simulink model "noloadwithcorrection"  (R2021a)
settings: Solver=VariableStepAuto  StartTime=0.0  StopTime=100  RelTol=1e-3
libraries: spsDCVoltageSourceLib x2, simulink x2, spsDCMachineLib x1, spsDiodeLib x1, spsGroundLib x1, spsIGBTDiodeLib x1, spspowerguiLib x1
settings Model: Creator=User  LastModifiedBy=User

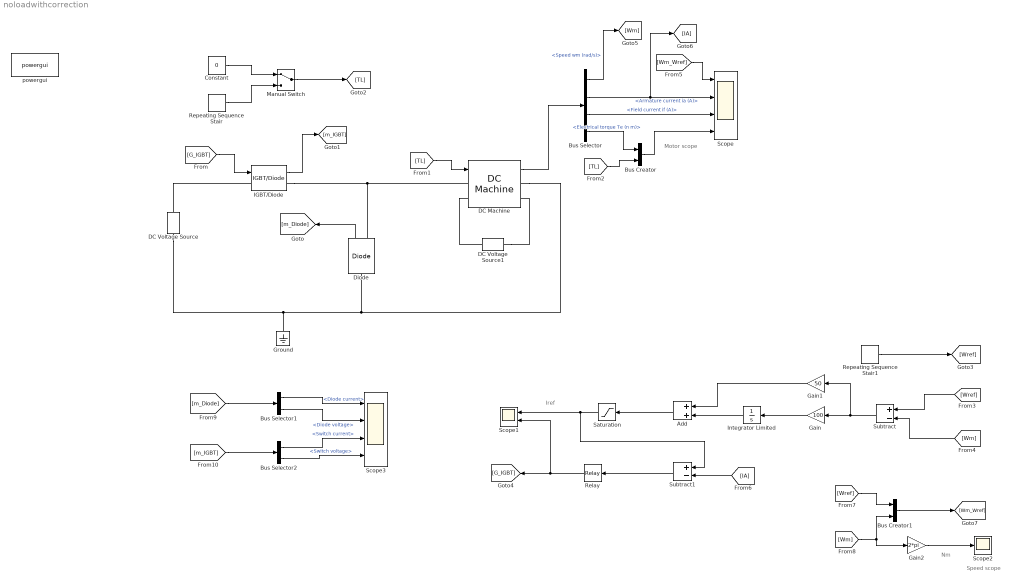
== system noloadwithcorrection ==
  note: Nm
  note: Speed scope
  note: Iref
  note: Motor scope
  Add : Sum
  Bus Creator : BusCreator  Inputs=2
  Bus Creator1 : BusCreator  Inputs=2
  Bus Selector : BusSelector  OutputSignals=Speed wm (rad/s),Armature current ia (A),Field current if (A),Electrical torque Te (n m)
  Bus Selector1 : BusSelector  OutputSignals=Diode current,Diode voltage
  Bus Selector2 : BusSelector  OutputSignals=Switch current,Switch voltage
  Constant : Constant  Value=0
  DC Machine : spsDCMachineLib/DC Machine  PresetModel=04: 10HP 240V 1750RPM Field:300V  MechanicalLoad=Torque TL  FieldType=Wound  ShowDetailedParameters=on  MeasurementBus=off  RLa=[1.086 0.01216]  RLf=[180 71.47]  Laf=0.6458  MachineConstant=Torque constant (N.m/A)  Ke=1.8  Kt=1.8  J=0.04251  Bm=0.003406  Tf=1.046  w0=1  Ifinit=1.66666666666667  TsPowergui=0  TsBlock=-1
  DC Voltage Source : spsDCVoltageSourceLib/DC Voltage Source  Amplitude=300  Measurements=None
  DC Voltage Source1 : spsDCVoltageSourceLib/DC Voltage Source  Amplitude=300  Measurements=None
  Diode : spsDiodeLib/Diode  Ron=0.001  Lon=0  Vf=0.8  IC=0  UseSnubber=0  Rs=500  Cs=250e-9  Measurements=on
  Gain : Gain  Gain=100
  Gain1 : Gain  Gain=50
  Gain2 : Gain  Gain=2*pi
  Ground : spsGroundLib/Ground  LConnTagsString=a
  IGBT/Diode : spsIGBTDiodeLib/IGBT//Diode  Ron=1e-3  Rs=1e5  Cs=inf  Measurements=on
  Integrator Limited : Integrator  LimitOutput=on  UpperSaturationLimit=1  LowerSaturationLimit=0
  Manual Switch : ManualSwitch
  Relay : Relay
  Repeating Sequence Stair : simulink/Sources/Repeating Sequence Stair  OutValues=[0 10 20 -2 15 0].'  tsamp=15  OutMin=[]  OutMax=[]  OutDataTypeStr=double  OutputDataTypeScalingMode=double  OutDataType=fixdt(0,8)  ConRadixGroup=Best Precision: Vector-wise  OutScaling=2^-12
  Repeating Sequence Stair1 : simulink/Sources/Repeating Sequence Stair  OutValues=[100 200 150 0].'  tsamp=10  OutMin=[]  OutMax=[]  OutDataTypeStr=double  OutputDataTypeScalingMode=double  OutDataType=fixdt(0,8)  ConRadixGroup=Best Precision: Vector-wise  OutScaling=2^-12
  Saturation : Saturate  UpperLimit=50  LowerLimit=0
  Scope : Scope  NumInputPorts=4
  Scope1 : Scope  NumInputPorts=2
  Scope2 : Scope
  Scope3 : Scope  NumInputPorts=4
  Subtract : Sum  Inputs=+-
  Subtract1 : Sum  Inputs=+-
  powergui : spspowerguiLib/powergui  Priority=1  SimulationMode=Discrete  SampleTime=0.0001  frequency=60  Iterations=50  frequencyindice=0  Pbase=100e6  ErrMax=1e-4  UnitsV=kV  UnitsW=MW  buscounter=0  FunctionMessages=off  echomessages=off  EnableUseOfTLC=off  CurrentSourceSwitches=off  DisableSnubberDevices=off  DisableRonSwitches=off  DisableVfSwitches=off  DisplayEquations=off  AutomaticDiscreteSolvers=off  SolverType=Tustin/Backward Euler (TBE)  Interpol=off  ExternalGateDelay=off  methode=off  Ts=100  x0status=blocks  SPID=on  SwTol=0  HookPort=off  NonlinearTolerance=1e-4  nMaxIteration=100  ContinueOnMaxIteration=off  RestoreLinks=warning  ResistiveCurrentMeasurement=off  Frange=[0:2:500]  Ylog=off  Xlog=on  ShowGrid=off  save=off  variable=ZData  structure=0  ZoomFFT=off  StartTime=0.0  cycles=1  DisplayStyle=1  fundamental=60  FreqAxis=off  MaxFrequency=1000  frequencyindicesteady=1  RmsSteady=1  display=off
  wires:
  [G_IGBT] -> IGBT/Diode/1
  Diode/1 -> [m_Diode]
  IGBT/Diode/1 -> [m_IGBT]
  [TL] -> DC Machine/1
  Constant/1 -> Manual Switch/1
  Repeating Sequence Stair/1 -> Manual Switch/2
  Manual Switch/1 -> [TL]
  DC Machine/1 -> Bus Selector/1
  Bus Selector/2 -> [IA], Scope/2  "<Armature current ia (A)>"
  Bus Selector/3 -> Scope/3  "<Field current if (A)>"
  Bus Selector/4 -> Bus Creator/1  "<Electrical torque Te (n m)>"
  [TL] -> Bus Creator/2
  Bus Creator/1 -> Scope/4
  Repeating Sequence Stair1/1 -> [Wref]
  [Wref] -> Subtract/1
  [Wm] -> Subtract/2
  Subtract/1 -> Gain1/1, Gain/1
  Gain/1 -> Integrator Limited/1
  Integrator Limited/1 -> Add/2
  Gain1/1 -> Add/1
  Add/1 -> Saturation/1
  Saturation/1 -> Subtract1/1, Scope1/1
  Relay/1 -> Scope1/2, [G_IGBT]
  Subtract1/1 -> Relay/1
  Bus Selector/1 -> [Wm]  "<Speed wm (rad/s)>"
  [Wm_Wref] -> Scope/1
  [IA] -> Subtract1/2
  [Wref] -> Bus Creator1/1
  [Wm] -> Bus Creator1/2, Gain2/1
  Bus Creator1/1 -> [Wm_Wref]
  Gain2/1 -> Scope2/1
  [m_Diode] -> Bus Selector1/1
  [m_IGBT] -> Bus Selector2/1
  Bus Selector1/1 -> Scope3/1  "<Diode current>"
  Bus Selector1/2 -> Scope3/2  "<Diode voltage>"
  Bus Selector2/1 -> Scope3/3  "<Switch current>"
  Bus Selector2/2 -> Scope3/4  "<Switch voltage>"
  connections:
  DC Voltage Source/RConn1 -- IGBT/Diode/LConn1
  IGBT/Diode/RConn1 -- DC Machine/LConn1 -- Diode/RConn1
  DC Voltage Source/LConn1 -- Ground/LConn1 -- DC Machine/RConn1 -- Diode/LConn1
  DC Voltage Source1/RConn1 -- DC Machine/LConn2
  DC Voltage Source1/LConn1 -- DC Machine/RConn2
